simulink model "System"  (R2023a)
settings: Solver=ode1be  StartTime=0.0  StopTime=10  FixedStep=0.001  RelTol=1e-3
settings Model: Creator=ycheb  LastModifiedBy=ycheb

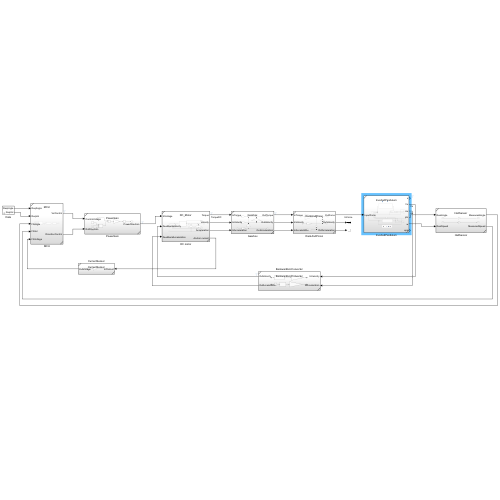
[thumbnail: Simulink's stored preview of the top-level diagram]
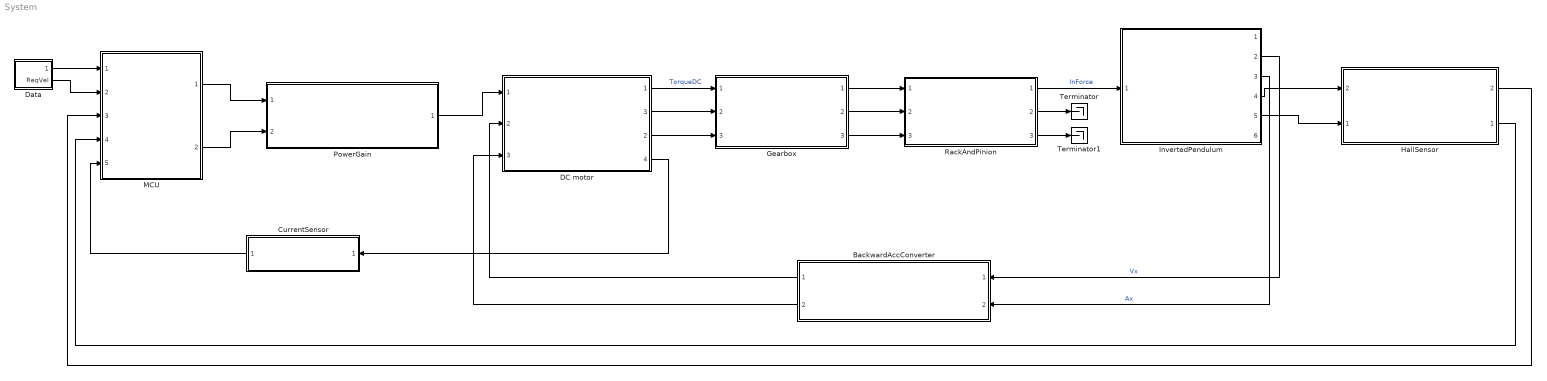
== system System ==
  BackwardAccConverter : Subsystem  ReferencedSubsystem=BackwardAccConverter
  CurrentSensor : Subsystem  ReferencedSubsystem=CurrentSensor
  DC motor : Subsystem  ReferencedSubsystem=DC_Motor
      settings: PortSchema="{\"entries\":[{\"content\":{\"sides\":[{\"content\":{\"connectorIds\":[\"In1\",\"In2\",\"In3\"]},\"type\":\"ConnectorPlacement.EquallySpacedRectSide\",\"uuid\":\"9bed3017-c50e-477b-981e-f56b8e2e9074\"},{\"content\":{\"connectorIds\":[\"Out1\",\"Out3\",\"Out2\",\"Out4\"],\"side\":\"RIGHT\"},\"type\":\"ConnectorPlacement.EquallySpacedRectSide\",\"uuid\":\"56040866-72b5-4c9e-836b-772424f49aa3\"},{\"content\":{\"side\":\"TOP\"},\"type\":\"ConnectorPlacement.EquallySpacedRectSide\",\"uuid\":\"8eaa70e9-c876-4040-8833-03b6a87fa78c\"}]},\"type\":\"ConnectorPlacement.EquallySpacedConnector\",\"uuid\":\"c559979a-d3c3-49f1-a55f-4b7abeb0eba0\"}],\"packageUris\":[\"http://schema.mathworks.com/mf0/Connector/R2020b\"],\"version\":\"1.0\"}"
  Data : Subsystem  mask{Angle=0, Vel=0}
      mask prompts: Angle "Requirenment angle"; Vel "Requirenment velocity"
  Gearbox : Subsystem  ReferencedSubsystem=Gearbox
  HallSensor : Subsystem  ReferencedSubsystem=HallSensor
      settings: PortSchema="{\"entries\":[{\"content\":{\"sides\":[{\"content\":{\"connectorIds\":[\"In2\",\"In1\"]},\"type\":\"ConnectorPlacement.EquallySpacedRectSide\",\"uuid\":\"805262f0-f66d-4bff-8129-d1c4f6a589e6\"},{\"content\":{\"connectorIds\":[\"Out2\",\"Out1\"],\"side\":\"RIGHT\"},\"type\":\"ConnectorPlacement.EquallySpacedRectSide\",\"uuid\":\"52da77b4-8929-4305-bc58-d5bd9d089017\"},{\"content\":{\"side\":\"TOP\"},\"type\":\"ConnectorPlacement.EquallySpacedRectSide\",\"uuid\":\"ce804b10-d076-4e17-a066-cbf164d447ac\"}]},\"type\":\"ConnectorPlacement.EquallySpacedConnector\",\"uuid\":\"f7301f1c-304a-4a03-b399-8f528c74926a\"}],\"packageUris\":[\"http://schema.mathworks.com/mf0/Connector/R2020b\"],\"version\":\"1.0\"}"
  InvertedPendulum : Subsystem  ReferencedSubsystem=InvertedPendulum
  MCU : Subsystem  ReferencedSubsystem=MCU
  PowerGain : Subsystem  ReferencedSubsystem=PowerGain
  RackAndPinion : Subsystem  ReferencedSubsystem=RackAndPinion
  Terminator : Terminator
  Terminator1 : Terminator
  wires:
  MCU/1 -> PowerGain/1
  MCU/2 -> PowerGain/2
  PowerGain/1 -> DC motor/1
  DC motor/2 -> Gearbox/3
  Gearbox/3 -> RackAndPinion/3
  Gearbox/2 -> RackAndPinion/2
  Gearbox/1 -> RackAndPinion/1
  RackAndPinion/1 -> InvertedPendulum/1  "InForce"
  RackAndPinion/2 -> Terminator/1
  RackAndPinion/3 -> Terminator1/1
  BackwardAccConverter/2 -> DC motor/3
  InvertedPendulum/4 -> HallSensor/2
  InvertedPendulum/5 -> HallSensor/1
  Data/1(ReqAngle) -> MCU/1
  Data/2(ReqVel) -> MCU/2
  HallSensor/2 -> MCU/3
  HallSensor/1 -> MCU/4
  DC motor/4 -> CurrentSensor/1
  CurrentSensor/1 -> MCU/5
  DC motor/1 -> Gearbox/1  "TorqueDC"
  DC motor/3 -> Gearbox/2
  InvertedPendulum/2 -> BackwardAccConverter/1  "Vx"
  InvertedPendulum/3 -> BackwardAccConverter/2  "Ax"
  BackwardAccConverter/1 -> DC motor/2

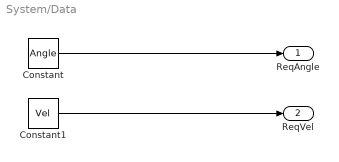
== system System/Data ==
  Constant : Constant  Value=Angle
  Constant1 : Constant  Value=Vel
  ReqAngle : Outport
  ReqVel : Outport  Port=2
  wires:
  Constant/1 -> ReqAngle/1
  Constant1/1 -> ReqVel/1
